simulink model "simpleDragTurbine_th"  (R2018b)
settings: Solver=VariableStepAuto  StartTime=0.0  StopTime=0  RelTol=1e-3
values from neighbouring files (symbols this model uses):
  V_flow = [1;0;0]    [simpleDragTurbine_ts.m]
  Vbody = [0;0;0]    [simpleDragTurbine_ts.m]
undefined symbols (not defined in the file or in its folder): euler
libraries: simpleDragTurbine_ul x1
settings Model: Creator=Ayaz  LastModifiedBy=asiddiq2

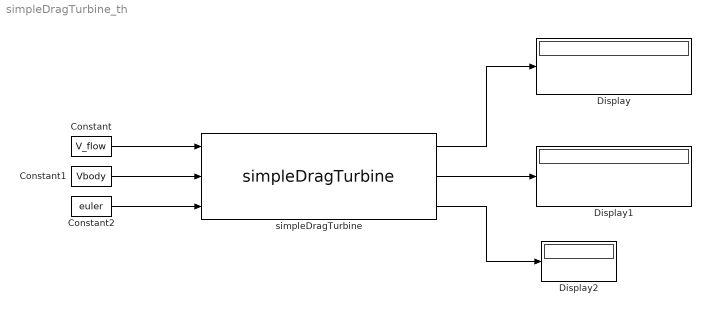
== system simpleDragTurbine_th ==
  Constant : Constant  Value=V_flow
  Constant1 : Constant  Value=Vbody
  Constant2 : Constant  Value=euler
  Display : Display
  Display1 : Display
  Display2 : Display
  simpleDragTurbine : simpleDragTurbine_ul/simpleDragTurbine  rho_fluid=rho_fluid  turb_struct=turbine
  wires:
  Constant/1 -> simpleDragTurbine/1
  Constant2/1 -> simpleDragTurbine/3
  Constant1/1 -> simpleDragTurbine/2
  simpleDragTurbine/1 -> Display/1
  simpleDragTurbine/2 -> Display1/1
  simpleDragTurbine/3 -> Display2/1
